simulink model "HVDVU_B6_adapted"  (R2024a)
settings: Solver=VariableStepAuto  StartTime=0.0  StopTime=0.04  RelTol=1e-3
libraries: spsThyristorLib x6, spsVoltageMeasurementLib x4, spsCurrentMeasurementLib x1, spsSeriesRLCBranchLib x1, spsThreePhaseSourceLib x1, spspowerguiLib x1
settings Model: Creator=bolt  LastModifiedBy=E370_
settings SolverCC: AlgebraicLoopSolver=TrustRegion
settings DebuggingCC: UnconnectedInputMsg=warning  UnconnectedOutputMsg=warning  UnconnectedLineMsg=warning
settings ModelReferenceCC: EnableRefExpFcnMdlSchedulingChecks=on
settings RTWCC: GPUComputeCapability=3.5

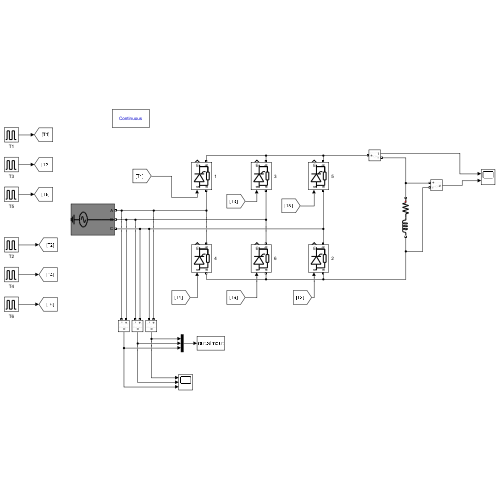
[thumbnail: Simulink's stored preview of the top-level diagram]
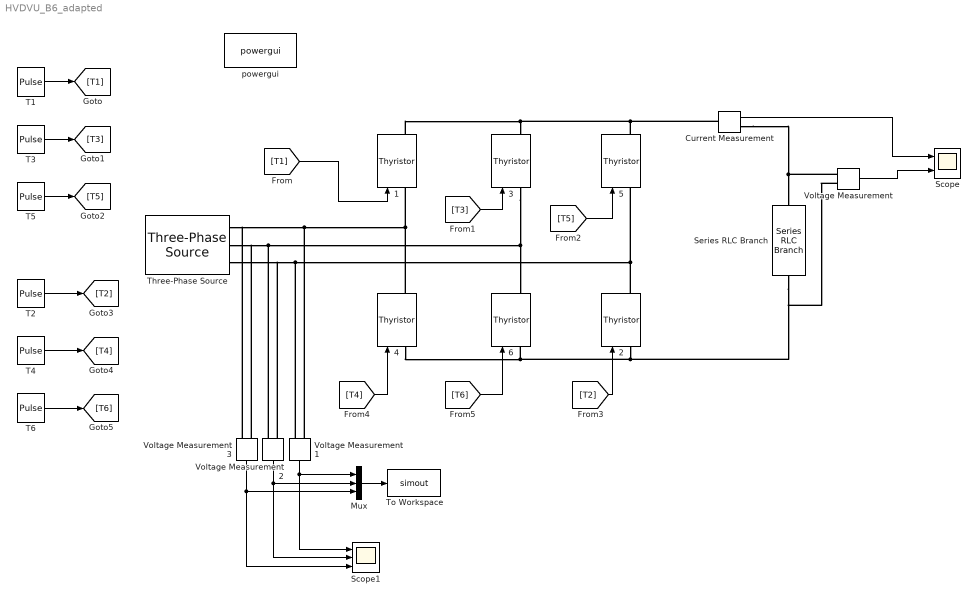
== system HVDVU_B6_adapted ==
  {1..6} (6 alike) : spsThyristorLib/Thyristor  Ron=0.001  Lon=0  Vf=0.8  IC=0  Rs=500  Cs=250e-9  Measurements=on
  Current Measurement : spsCurrentMeasurementLib/Current Measurement  PhasorSimulation=off  OutputType=Complex  PSBequivalent=0
  Mux : Mux  Inputs=3
  Scope : Scope  NumInputPorts=2
  Scope1 : Scope  NumInputPorts=3
  Series RLC Branch : spsSeriesRLCBranchLib/Series RLC Branch  LConnTagsString=__new0  RConnTagsString=__new0  BranchType=RL  Resistance=5000  Inductance=100e-3  SetiL0=off  InitialCurrent=0  Capacitance=1e-6  Setx0=off  InitialVoltage=0  Measurements=None
  T1 : DiscretePulseGenerator  PulseType=Time based  Period=0.02  PulseWidth=5  PhaseDelay=0.00334
  T2 : DiscretePulseGenerator  PulseType=Time based  Period=0.02  PulseWidth=5  PhaseDelay=0.00668
  T3 : DiscretePulseGenerator  PulseType=Time based  Period=0.02  PulseWidth=5  PhaseDelay=0.01
  T4 : DiscretePulseGenerator  PulseType=Time based  Period=0.02  PulseWidth=5  PhaseDelay=0.00334+0.01
  T5 : DiscretePulseGenerator  PulseType=Time based  Period=0.02  PulseWidth=5  PhaseDelay=0.01+0.00668
  T6 : DiscretePulseGenerator  PulseType=Time based  Period=0.02  PulseWidth=5
  Three-Phase Source : spsThreePhaseSourceLib/Three-Phase Source  InternalConnection=Yg  VoltagePhases=off  Voltage=100  PhaseAngle=0  Voltage_phases=[25e3 25e3 25e3]/sqrt(3)  PhaseAngles_phases=[0 -120 +120]  Frequency=50  NonIdealSource=off  SpecifyImpedance=off  Resistance=0.8929  Inductance=16.58e-3  ShortCircuitLevel=100e6  BaseVoltage=25e3  XRratio=7  BusType=swing  Pref=10e3  Qref=0  Prefabc=[10e3, 10e3, 10e3]  Qrefabc=[0, 0, 0]  Qmin=-inf  Qmax=inf
  To Workspace : ToWorkspace  VariableName=simout  SaveFormat=Timeseries  SampleTime=-1
  Voltage Measurement{,1..3} (4 alike) : spsVoltageMeasurementLib/Voltage Measurement  PhasorSimulation=off  OutputType=Complex  PSBequivalent=0
  powergui : spspowerguiLib/powergui  Priority=1  SimulationMode=Continuous  SampleTime=50e-6  frequency=60  Iterations=50  frequencyindice=50  Pbase=100e6  ErrMax=1e-4  UnitsV=kV  UnitsW=MW  buscounter=0  FunctionMessages=off  echomessages=off  EnableUseOfTLC=off  CurrentSourceSwitches=off  DisableSnubberDevices=off  DisableRonSwitches=off  DisableVfSwitches=off  DisplayEquations=off  AutomaticDiscreteSolvers=off  SolverType=Tustin/Backward Euler (TBE)  Interpol=off  ExternalGateDelay=off  methode=off  Ts=100  x0status=blocks  SPID=on  SwTol=0  HookPort=off  NonlinearTolerance=1e-4  nMaxIteration=100  ContinueOnMaxIteration=off  RestoreLinks=warning  ResistiveCurrentMeasurement=off  Frange=[0:2:500]  Ylog=off  Xlog=on  ShowGrid=off  save=off  variable=ZData  structure=0  ZoomFFT=off  StartTime=0.0  cycles=1  DisplayStyle=1  fundamental=60  FreqAxis=off  MaxFrequency=1000  frequencyindicesteady=1  RmsSteady=1  display=off
  wires:
  T1/1 -> [T1]
  T3/1 -> [T3]
  T5/1 -> [T5]
  T2/1 -> [T2]
  T4/1 -> [T4]
  T6/1 -> [T6]
  [T1] -> 1/1
  [T3] -> 3/1
  [T5] -> 5/1
  [T2] -> 2/1
  Voltage Measurement/1 -> Scope/2
  Current Measurement/1 -> Scope/1
  [T4] -> 4/1
  [T6] -> 6/1
  Voltage Measurement3/1 -> Mux/3, Scope1/3
  Voltage Measurement2/1 -> Mux/2, Scope1/2
  Voltage Measurement1/1 -> Mux/1, Scope1/1
  Mux/1 -> To Workspace/1
  connections:
  4/RConn1 -- Voltage Measurement1/LConn1 -- Voltage Measurement3/LConn2 -- Three-Phase Source/RConn1 -- 1/LConn1
  3/LConn1 -- Voltage Measurement2/LConn2 -- Voltage Measurement3/LConn1 -- Three-Phase Source/RConn2 -- 6/RConn1
  2/RConn1 -- Voltage Measurement1/LConn2 -- Voltage Measurement2/LConn1 -- Three-Phase Source/RConn3 -- 5/LConn1
  5/RConn1 -- 1/RConn1 -- 3/RConn1 -- Current Measurement/LConn1
  4/LConn1 -- Voltage Measurement/LConn2 -- Series RLC Branch/RConn1 -- 2/LConn1 -- 6/LConn1
  Current Measurement/RConn1 -- Voltage Measurement/LConn1 -- Series RLC Branch/LConn1
